simulink model "androidSerialPWMServoSend_Arduino"  (R2019a)
settings: Solver=ode3  StartTime=0.0  StopTime=inf  RelTol=1e-3  EnableMultiTasking=on
libraries: arduinolib x10
settings Model: ExtModeTrigDuration=2  Creator=The MathWorks, Inc.  LastModifiedBy=Alireza
settings DataIOCC: LimitDataPoints=on  SaveFormat=Array  ReturnWorkspaceOutputs=off
settings OptimizationCC: DefaultUnderspecifiedDataType=single  ExpressionDepthLimit=2147483647  LifeSpan=Inf  MaxStackSize=64
settings DebuggingCC: UnderspecifiedInitializationDetection=Classic  MergeDetectMultiDrivingBlocksExec=none  InheritedTsInSrcMsg=none  ParameterPrecisionLossMsg=none  FcnCallInpInsideContextMsg=warning  AllowSymbolicDim=off  StateNameClashWarn=warning  SymbolicDimsDataTypeCodeGenerationDiagnostic=none  SFUnexpectedBacktrackingDiag=warning  SFNoUnconditionalDefaultTransitionDiag=warning  SFExecutionAtInitializationDiag=none  ArithmeticOperatorsInVariantConditions=warning
settings HardwareCC: ProdBitPerInt=16  ProdBitPerPointer=16  ProdBitPerSizeT=16  ProdBitPerPtrDiffT=16  ProdLargestAtomicFloat=None  ProdWordSize=8  ProdHWDeviceType=Atmel->AVR
settings ModelReferenceCC: PropagateSignalLabelsOutOfModel=off
settings SFSimCC: SimUseLocalCustomCode=off  MATLABDynamicMemAlloc=off
settings RTWCC: SystemTargetFile=ert.tlc  HardwareBoard=Arduino Mega 2560  TemplateMakefile=ert_default_tmf  GenerateReport=on  RTWVerbose=off  RTWUseLocalCustomCode=off  Toolchain=Arduino AVR  BuildConfiguration=Faster Runs  LaunchReport=on
settings CodeAppCC: ForceParamTrailComments=on  OperatorAnnotations=on  StateflowObjectComments=on  MATLABSourceComments=on
settings ERTTargetCC: MultiwordLength=2048  ERTCustomFileBanners=off  SupportContinuousTime=on  SupportNonInlinedSFcns=on  RemoveResetFunc=off  SupportVariableSizeSignals=on  ModelStepFunctionPrototypeControlCompliant=off  ExtModeStaticAllocSize=2048
settings ConfigComp: CovMetricSettings=dw  CovHtmlReporting=on  CovSaveCumulativeToWorkspaceVar=on  CovSaveSingleToWorkspaceVar=on  CovExternalEMLEnable=off  CovSFcnEnable=off

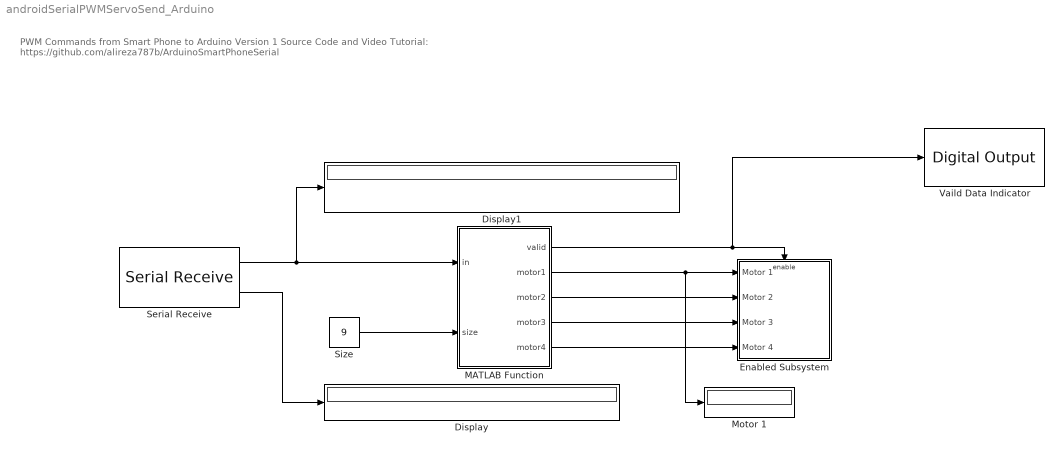
== system androidSerialPWMServoSend_Arduino ==
  note: PWM Commands from Smart Phone to Arduino Version 1
      | Source Code and Video Tutorial:
      | https://github.com/alireza787b/ArduinoSmartPhoneSerial
  Display : Display
  Display1 : Display
  Enabled Subsystem : Subsystem  TreatAsAtomicUnit=on
  MATLAB Function : MATLAB Function  TreatAsAtomicUnit=on
  Motor 1 : Display
  Serial Receive : arduinolib/Serial Receive  isARMArch=off  portNumber=1  DataType=uint8  Datalength=9  SampleTime=0.01  showOutStatus=on  blockPlatform=arduino
      settings: SourceProductBaseCode=ARDUINO
  Size : Constant  Value=9  OutDataTypeStr=uint8
  Vaild Data Indicator : arduinolib/Digital Output  pinNumber=13  Direction=output  blockPlatform=arduino
  wires:
  Size/1 -> MATLAB Function/2(size)
  MATLAB Function/2(motor1) -> Motor 1/1, Enabled Subsystem/1(Motor 1)
  MATLAB Function/3(motor2) -> Enabled Subsystem/2(Motor 2)
  MATLAB Function/4(motor3) -> Enabled Subsystem/3(Motor 3)
  MATLAB Function/5(motor4) -> Enabled Subsystem/4(Motor 4)
  Serial Receive/1 -> Display1/1, MATLAB Function/1(in)
  Serial Receive/2 -> Display/1
  MATLAB Function/1(valid) -> Vaild Data Indicator/1, Enabled Subsystem/Enable

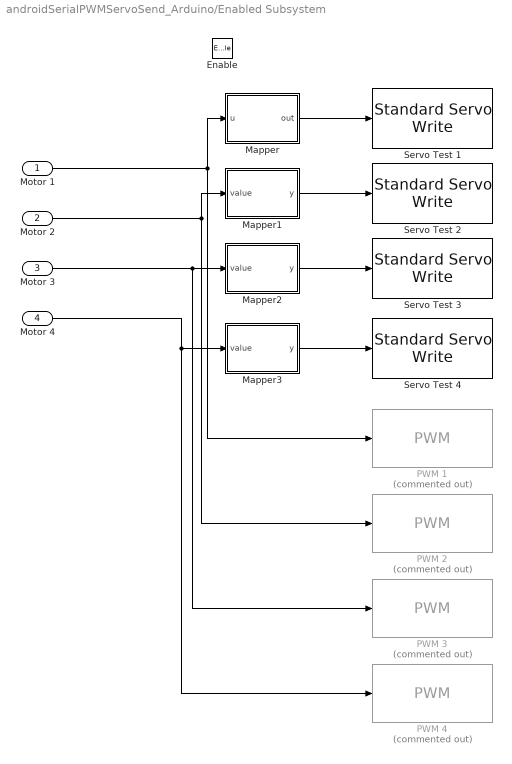
== system androidSerialPWMServoSend_Arduino/Enabled Subsystem ==
  Motor 1 : Inport
  Motor 2 : Inport  Port=2
  Motor 3 : Inport  Port=3
  Motor 4 : Inport  Port=4
  Enable : EnablePort  StatesWhenEnabling=reset  ShowOutputPort=on
  Mapper : MATLAB Function  TreatAsAtomicUnit=on
  Mapper1 : MATLAB Function  TreatAsAtomicUnit=on
  Mapper2 : MATLAB Function  TreatAsAtomicUnit=on
  Mapper3 : MATLAB Function  TreatAsAtomicUnit=on
  PWM 1 : arduinolib/PWM  Commented=on  pinNumber=9  frequencyType=Default  desiredFrequency=490.2  achievableFrequency=490.2
  PWM 2 : arduinolib/PWM  Commented=on  pinNumber=10  frequencyType=Default  desiredFrequency=490.2  achievableFrequency=490.2
  PWM 3 : arduinolib/PWM  Commented=on  pinNumber=3  frequencyType=Default  desiredFrequency=490.2  achievableFrequency=490.2
  PWM 4 : arduinolib/PWM  Commented=on  pinNumber=4  frequencyType=Default  desiredFrequency=490.2  achievableFrequency=490.2
  Servo Test 1 : arduinolib/Standard Servo Write  pinNumber=9  ServoIndex=0  blockPlatform=arduino
  Servo Test 2 : arduinolib/Standard Servo Write  pinNumber=10  ServoIndex=1  blockPlatform=arduino
  Servo Test 3 : arduinolib/Standard Servo Write  pinNumber=5  ServoIndex=2  blockPlatform=arduino
  Servo Test 4 : arduinolib/Standard Servo Write  pinNumber=6  ServoIndex=3  blockPlatform=arduino
  wires:
  Mapper/1(out) -> Servo Test 1/1
  Motor 1/1 -> PWM 1/1, Mapper/1(u)
  Motor 2/1 -> PWM 2/1, Mapper1/1(value)
  Mapper1/1(y) -> Servo Test 2/1
  Mapper3/1(y) -> Servo Test 4/1
  Motor 3/1 -> PWM 3/1, Mapper2/1(value)
  Mapper2/1(y) -> Servo Test 3/1
  Motor 4/1 -> PWM 4/1, Mapper3/1(value)

== matlab function androidSerialPWMServoSend_Arduino/Enabled Subsystem/Mapper ==
  data: u input; out output
function out= mapper(u)
value = cast(u,'single');
fromLow = 0;
fromHigh = 255;
toLow = 20;
toHigh = 160;
y = (value - fromLow) .* (toHigh - toLow) ./ (fromHigh - fromLow) + toLow;
out = cast(y,'uint8');
end

== matlab function androidSerialPWMServoSend_Arduino/MATLAB Function ==
  data: in input; valid output; size input; motor1 output; motor2 output; motor3 output; motor4 output
function [valid,motor1,motor2,motor3,motor4] = dataCheck(in,size)
if(in(1) == 68 && in(2) == 65 && in(3) == 84 && in(4) == 65 && in(size) == 10)
    valid = true;
    motor1 = in(5);
    motor2 = in(6);
    motor3 = in(7);
    motor4 = in(8);
else 
    valid = false;
    motor1 = uint8(0);
    motor2 = uint8(0);
    motor3 = uint8(0);
    motor4 = uint8(0);
end

end

== matlab function androidSerialPWMServoSend_Arduino/Enabled Subsystem/Mapper1 ==
  data: value input; y output
function y = mapper(value)
fromLow = 0;
fromHigh = 255;
toLow = 20;
toHigh = 160;
y = (value - fromLow) .* (toHigh - toLow) ./ (fromHigh - fromLow) + toLow;
end

== matlab function androidSerialPWMServoSend_Arduino/Enabled Subsystem/Mapper2 ==
  data: value input; y output
function y = mapper(value)
fromLow = 0;
fromHigh = 255;
toLow = 20;
toHigh = 160;
y = (value - fromLow) .* (toHigh - toLow) ./ (fromHigh - fromLow) + toLow;
end

== matlab function androidSerialPWMServoSend_Arduino/Enabled Subsystem/Mapper3 ==
  data: value input; y output
function y = mapper(value)
fromLow = 0;
fromHigh = 255;
toLow = 20;
toHigh = 160;
y = (value - fromLow) .* (toHigh - toLow) ./ (fromHigh - fromLow) + toLow;
end
